simulink model "Paper_Simulation"  (R2020a)
settings: Solver=VariableStepAuto  StartTime=0.0  StopTime=10.0  RelTol=1e-3
model workspace (MAT data in the model file):
  Wo = 1
undefined symbols (not defined in the file): fdesignblkfcn, gcbh, T1, T2, Tf
libraries: eeSinusoidalMeasurementV2 x1, simulink x1
settings Model: Creator=Ayush Agrawal  LastModifiedBy=Ayush Agrawal

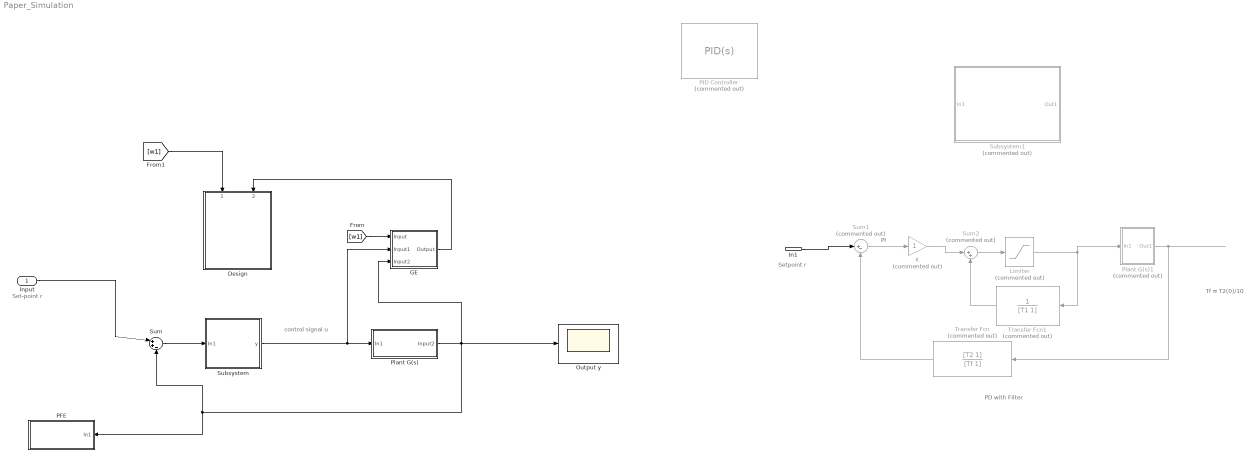
== system Paper_Simulation ==
  note: control signal
      |         u
  note: Set-point r
  note: Setpoint r
  note: PI
  note: PD with Filter
  note: Tf = T2(0)/10
  Input : Inport
  In1 : Inport  Port=2
  Design : Subsystem  mask{a=1.5}
  GE : Subsystem
  K : Gain  Commented=on
  Limiter : Saturate  Commented=on
  Output y : Scope
  PFE : Subsystem
  PID Controller : simulink/Continuous/PID Controller  Commented=on  Controller=PID  Form=Parallel  TimeDomain=Continuous-time  UseExternalTs=off  SampleTime=-1  IntegratorMethod=Forward Euler  FilterMethod=Forward Euler  ControllerParametersSource=internal  P=1  I=1  D=0  UseFilter=on  N=100  TunerSelectOption=Transfer Function Based (PID Tuner App)  InitialConditionSource=internal  InitialConditionForIntegrator=0  InitialConditionForFilter=0  DifferentiatorICPrevScaledInput=0  ExternalReset=none  TrackingMode=off  Kt=1  LimitOutput=off  UpperSaturationLimit=inf  LowerSaturationLimit=-inf  LinearizeAsGain=on  AntiWindupMode=none  Kb=1  POutMin=[]  POutMax=[]  IOutMin=[]  IOutMax=[]  DOutMin=[]  DOutMax=[]  NOutMin=[]  NOutMax=[]  SumOutMin=[]  SumOutMax=[]  SaturationOutMin=[]  SaturationOutMax=[]  PParamMin=[]  PParamMax=[]  IParamMin=[]  IParamMax=[]  DParamMin=[]  DParamMax=[]  NParamMin=[]  NParamMax=[]  KbParamMin=[]  KbParamMax=[]  KtParamMin=[]  KtParamMax=[]  KbOutMin=[]  KbOutMax=[]  KtOutMin=[]  KtOutMax=[]  IntegratorOutMin=[]  IntegratorOutMax=[]  FilterOutMin=[]  FilterOutMax=[]  SumI1OutMin=[]  SumI1OutMax=[]  SumI2OutMin=[]  SumI2OutMax=[]  SumI3OutMin=[]  SumI3OutMax=[]  SumI4OutMin=[]  SumI4OutMax=[]  SumDOutMin=[]  SumDOutMax=[]  DifferentiatorOutMin=[]  DifferentiatorOutMax=[]  FilterDiffOutCoefMin=[]  FilterDiffOutCoefMax=[]  ReciprocalOutMin=[]  ReciprocalOutMax=[]  SumDenOutMin=[]  SumDenOutMax=[]  SumNumOutMin=[]  SumNumOutMax=[]  DivideOutMin=[]  DivideOutMax=[]  UdiffTsProdOutMin=[]  UdiffTsProdOutMax=[]  NTsProdOutMin=[]  NTsProdOutMax=[]  UintegralTsProdOutMin=[]  UintegralTsProdOutMax=[]  UngainTsProdOutMin=[]  UngainTsProdOutMax=[]  IntegratorContinuousStateAttributes=''  IntegratorStateMustResolveToSignalObject=off  IntegratorRTWStateStorageClass=Auto  FilterContinuousStateAttributes=''  FilterStateMustResolveToSignalObject=off  FilterRTWStateStorageClass=Auto  ParallelPVariant=InternalParameters  IdealPVariant=Disabled  IVariant=InternalParameters  DVariant=InternalParameters  IntegratorVariant=Continuous  SatVariant=Disabled  AWVariant=Passthrough  PCopyVariant=Disabled  TRVariant=Disabled  FdbkBlocksVariant=Forward  IdealPFdbkVariant=Disabled  SatFdbkVariant=Disabled  DerivativeFilterVariant=ContFilter  NVariant=InternalParameters  NCopyVariant=Disabled  FilterICVariant=InternalICsFilter  IntegratorICVariant=InternalICs  ExternalResetVariant=Disabled  TRSumVariant=Passthrough  SumFdbkVariant=Disabled  SumVariant=Sum_PID  TsampFilterVariant=InternalTs  TsampNgainVariant=Passthrough  TsampIntegralVariant=Passthrough
  Plant G(s) : Subsystem
  Plant G(s)1 : Subsystem  Commented=on
  Subsystem : Subsystem  mask{Ti=0, r=0}
  Subsystem1 : Subsystem  Commented=on
  Sum : Sum  Inputs=|++-
  Sum1 : Sum  Commented=on  Inputs=|+-
  Sum2 : Sum  Commented=on  Inputs=|++
  Transfer Fcn : TransferFcn  Commented=on  Numerator=[T2 1]  Denominator=[Tf 1]
  Transfer Fcn1 : TransferFcn  Commented=on  Denominator=[T1 1]
  wires:
  Plant G(s)/1(Input2) -> GE/3(Input2), Output y/1, Sum/3, PFE/1(In1)
  ? -> Sum/2
  Input/1 -> Sum/1
  Sum2/1 -> Limiter/1
  In1/1 -> Sum1/1
  Plant G(s)1/1(Out1) -> Transfer Fcn/1
  Limiter/1 -> Transfer Fcn1/1, Plant G(s)1/1(In1)
  Sum1/1 -> K/1
  Transfer Fcn/1 -> Sum1/2
  K/1 -> Sum2/1
  Transfer Fcn1/1 -> Sum2/2
  [w1] -> GE/1(Input)
  GE/1(Output) -> Design/2(Plant Gain Amplitude)
  [w1] -> Design/1(PFE O/P frequency)
  Subsystem/1(y) -> GE/2(Input1), Plant G(s)/1(In1)
  Sum/1 -> Subsystem/1(In1)

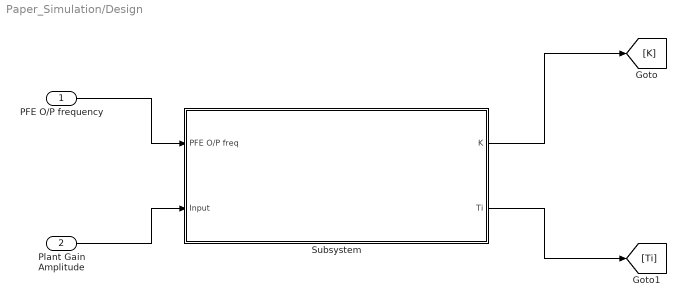
== system Paper_Simulation/Design ==
  PFE O/P frequency : Inport
  Plant Gain Amplitude : Inport  Port=2
  Subsystem : Subsystem
  wires:
  PFE O/P frequency/1 -> Subsystem/1(PFE O/P freq)
  Plant Gain Amplitude/1 -> Subsystem/2(Input)
  Subsystem/1(K) -> [K]
  Subsystem/2(Ti) -> [Ti]

== system Paper_Simulation/GE ==
  Input : Inport
  Input1 : Inport  Port=2
  Input2 : Inport  Port=3
  Amplitude Estimator : Subsystem
  Output : Outport
  wires:
  Input1/1 -> Amplitude Estimator/1(In1)
  Input/1 -> Amplitude Estimator/2(Input)
  Amplitude Estimator/1(Output) -> Output/1

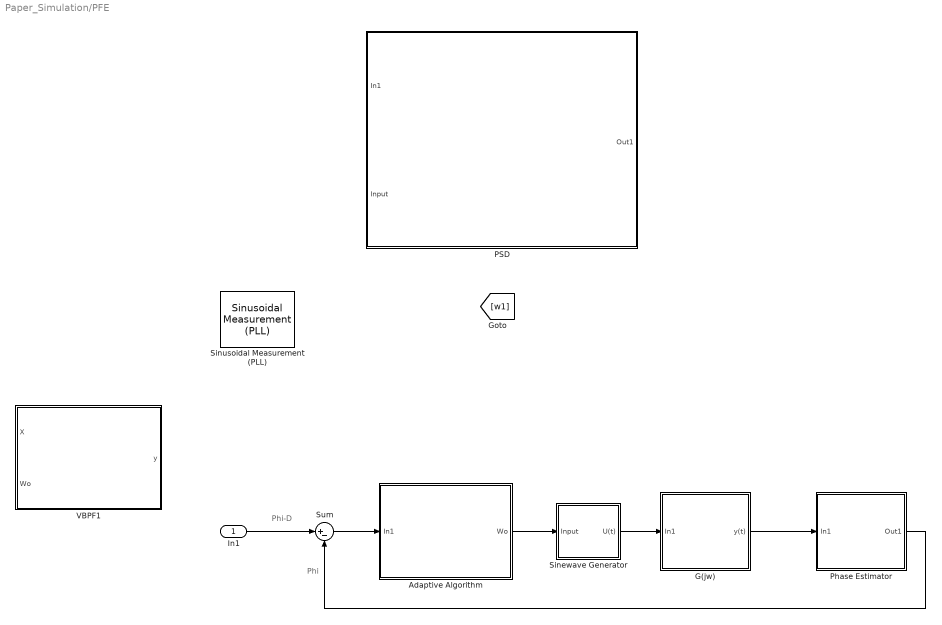
== system Paper_Simulation/PFE ==
  note: Phi
  note: Phi-D
  In1 : Inport
  Adaptive Algorithm : Subsystem
  G(jw) : Subsystem
  PSD : Subsystem
  Phase Estimator : Subsystem
  Sinewave Generator : Subsystem
  Sinusoidal Measurement (PLL) : eeSinusoidalMeasurementV2/Sinusoidal Measurement (PLL)  Ki_PD=1000  Kp_LF=400  Ki_LF=20000  F0=60  Theta0=0  Mag0=1  Ts=-1
      settings: SourceProductBaseCode=PS
  Sum : Sum  Inputs=|+-
  VBPF1 : Subsystem
  wires:
  In1/1 -> Sum/1
  Sum/1 -> Adaptive Algorithm/1(In1)
  Adaptive Algorithm/1(Wo) -> Sinewave Generator/1(Input)
  Sinewave Generator/1(U(t)) -> G(jw)/1(In1)
  G(jw)/1(y(t)) -> Phase Estimator/1(In1)
  Phase Estimator/1(Out1) -> Sum/2

== system Paper_Simulation/Plant G(s) ==
  In1 : Inport
  Input2 : Outport
  wires:
  In1/1 -> Input2/1

== system Paper_Simulation/Plant G(s)1 ==
  In1 : Inport
  Out1 : Outport
  wires:
  In1/1 -> Out1/1

== system Paper_Simulation/Subsystem ==
  In1 : Inport
  Controller : Subsystem  mask{Td=Ti*r, Tf=0, T1=Ti/2, T2=Ti/2}
  y : Outport
  wires:
  Controller/1(y) -> y/1
  In1/1 -> Controller/1(In1)

== system Paper_Simulation/Subsystem1 ==
  In1 : Inport
  Out1 : Outport
  wires:
  In1/1 -> Out1/1

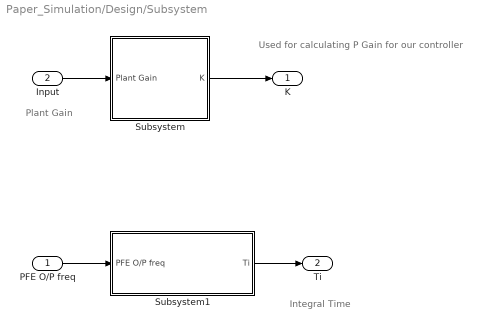
== system Paper_Simulation/Design/Subsystem ==
  note: Used for calculating P Gain for our controller
  note: Integral Time
  note: Plant Gain
  PFE O/P freq : Inport
  Input : Inport  Port=2
  Subsystem : Subsystem
  Subsystem1 : Subsystem
  K : Outport
  Ti : Outport  Port=2
  wires:
  Input/1 -> Subsystem/1(Plant Gain)
  Subsystem/1(K) -> K/1
  PFE O/P freq/1 -> Subsystem1/1(PFE O/P freq)
  Subsystem1/1(Ti) -> Ti/1

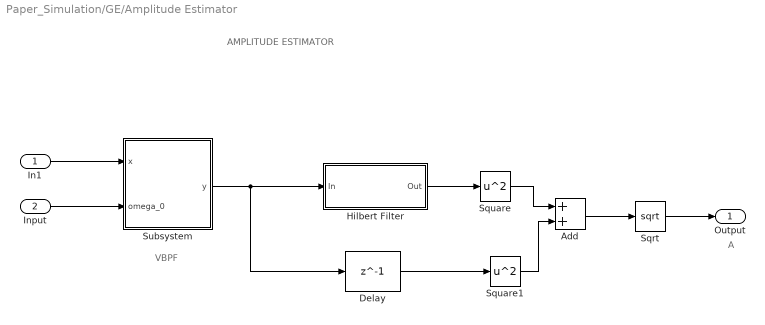
== system Paper_Simulation/GE/Amplitude Estimator ==
  note: A
  note: AMPLITUDE ESTIMATOR
  note: VBPF
  In1 : Inport
  Input : Inport  Port=2
  Add : Sum
  Delay : Delay  DelayLength=1  InitialCondition=0  UseCircularBuffer=on
  Hilbert Filter : Subsystem  DialogController=fdesignblkfcn  InitFcn=fdesignblkfcn(gcbh, {'InitFcn'});  mask(Hilbert Filter){}
      mask help: Design a Hilbert filter
      settings: CopyFcn=fdesignblkfcn(gcbh, {'CopyFcn'});
      mask Help: helpview(mapfilelocation('dsp'), 'dsphilbertfilter');
      mask Display: disp('Hilbert')
  Sqrt : Sqrt  SaturateOnIntegerOverflow=on
  Square : Math  Operator=square  SaturateOnIntegerOverflow=on
  Square1 : Math  Operator=square  SaturateOnIntegerOverflow=on
  Subsystem : Subsystem
  Output : Outport
  wires:
  Input/1 -> Subsystem/2(omega_0)
  In1/1 -> Subsystem/1(x)
  Subsystem/1(y) -> Delay/1, Hilbert Filter/1(In)
  Hilbert Filter/1(Out) -> Square/1
  Delay/1 -> Square1/1
  Square/1 -> Add/1
  Square1/1 -> Add/2
  Add/1 -> Sqrt/1
  Sqrt/1 -> Output/1

== system Paper_Simulation/PFE/Adaptive Algorithm ==
  In1 : Inport
  Wo : Outport
  wires:
  In1/1 -> Wo/1

== system Paper_Simulation/PFE/G(jw) ==
  In1 : Inport
  y(t) : Outport

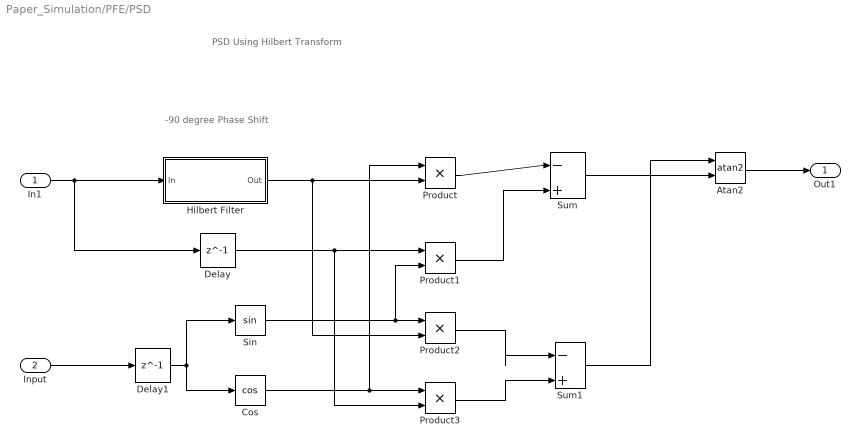
== system Paper_Simulation/PFE/PSD ==
  note: -90 degree Phase Shift
  note: PSD Using Hilbert Transform
  In1 : Inport
  Input : Inport  Port=2
  Atan2 : Trigonometry  Operator=atan2
  Cos : Trigonometry  Operator=cos
  Delay : Delay  DelayLength=1
  Delay1 : Delay  DelayLength=1
  Hilbert Filter : Subsystem  DialogController=fdesignblkfcn  InitFcn=fdesignblkfcn(gcbh, {'InitFcn'});  mask(Hilbert Filter){}
      mask help: Design a Hilbert filter
      settings: CopyFcn=fdesignblkfcn(gcbh, {'CopyFcn'});
      mask Help: helpview(mapfilelocation('dsp'), 'dsphilbertfilter');
      mask Display: disp('Hilbert')
  Product{,1..3} (4 alike) : Product
  Sin : Trigonometry
  Sum : Sum  Inputs=|-+
  Sum1 : Sum  Inputs=|-+
  Out1 : Outport
  wires:
  In1/1 -> Delay/1, Hilbert Filter/1(In)
  Hilbert Filter/1(Out) -> Product2/2, Product/2
  Input/1 -> Delay1/1
  Delay1/1 -> Sin/1, Cos/1
  Sin/1 -> Product1/2, Product2/1
  Cos/1 -> Product/1, Product3/1
  Delay/1 -> Product3/2, Product1/1
  Product/1 -> Sum/1
  Product1/1 -> Sum/2
  Atan2/1 -> Out1/1
  Sum/1 -> Atan2/2
  Product2/1 -> Sum1/1
  Product3/1 -> Sum1/2
  Sum1/1 -> Atan2/1

== system Paper_Simulation/PFE/Phase Estimator ==
  In1 : Inport
  Out1 : Outport
  wires:
  In1/1 -> Out1/1

== system Paper_Simulation/PFE/Sinewave Generator ==
  Input : Inport
  U(t) : Outport

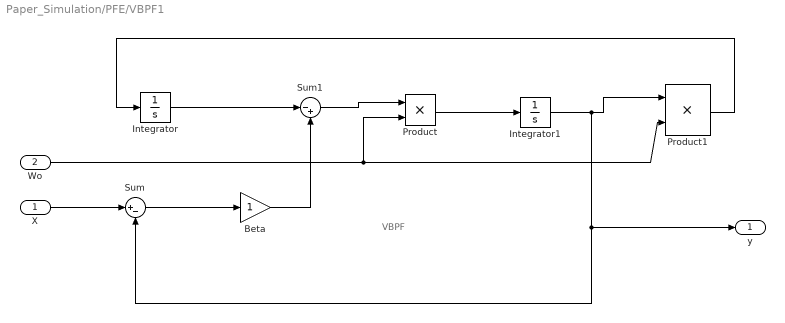
== system Paper_Simulation/PFE/VBPF1 ==
  note: VBPF
  X : Inport
  Wo : Inport  Port=2
  Beta : Gain
  Integrator : Integrator
  Integrator1 : Integrator
  Product : Product
  Product1 : Product
  Sum : Sum  Inputs=|+-
  Sum1 : Sum  Inputs=|-+
  y : Outport
  wires:
  X/1 -> Sum/1
  Sum/1 -> Beta/1
  Integrator/1 -> Sum1/1
  Beta/1 -> Sum1/2
  Sum1/1 -> Product/1
  Wo/1 -> Product1/2, Product/2
  Product/1 -> Integrator1/1
  Integrator1/1 -> Product1/1, Sum/2, y/1
  Product1/1 -> Integrator/1

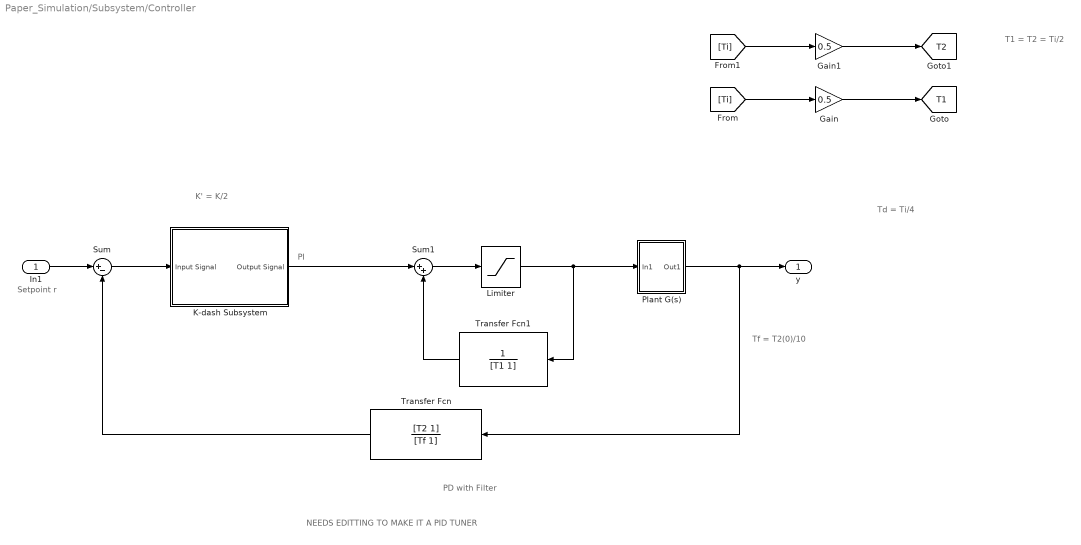
== system Paper_Simulation/Subsystem/Controller ==
  note: K' = K/2
  note: Td = Ti/4
  note: T1 = T2 = Ti/2
  note: NEEDS EDITTING TO MAKE IT A PID TUNER
  note: PI
  note: PD with Filter
  note: Setpoint r
  note: Tf = T2(0)/10
  In1 : Inport
  Gain : Gain  Gain=0.5
  Gain1 : Gain  Gain=0.5
  K-dash Subsystem : Subsystem
  Limiter : Saturate
  Plant G(s) : Subsystem
  Sum : Sum  Inputs=|+-
  Sum1 : Sum  Inputs=|++
  Transfer Fcn : TransferFcn  Numerator=[T2 1]  Denominator=[Tf 1]
  Transfer Fcn1 : TransferFcn  Denominator=[T1 1]
  y : Outport
  tag scope: T1=global, T2=global
  wires:
  Sum/1 -> K-dash Subsystem/1(Input Signal)
  Sum1/1 -> Limiter/1
  Limiter/1 -> Transfer Fcn1/1, Plant G(s)/1(In1)
  Transfer Fcn1/1 -> Sum1/2
  In1/1 -> Sum/1
  K-dash Subsystem/1(Output Signal) -> Sum1/1
  Plant G(s)/1(Out1) -> Transfer Fcn/1, y/1
  Transfer Fcn/1 -> Sum/2
  [Ti] -> Gain/1
  Gain/1 -> [T1]
  Gain1/1 -> [T2]
  [Ti] -> Gain1/1

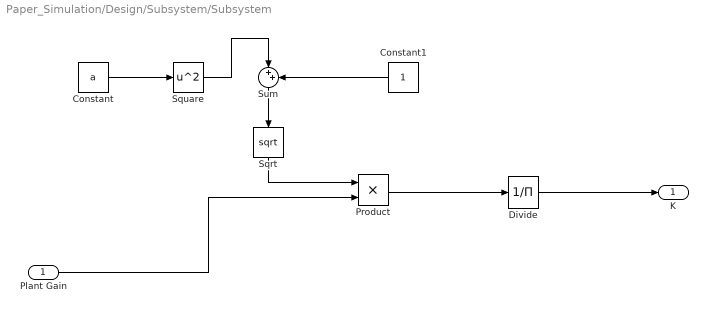
== system Paper_Simulation/Design/Subsystem/Subsystem ==
  Plant Gain : Inport
  Constant : Constant  Value=a
  Constant1 : Constant
  Divide : Product  Inputs=/
  Product : Product
  Sqrt : Sqrt  SaturateOnIntegerOverflow=on
  Square : Math  Operator=square  SaturateOnIntegerOverflow=on
  Sum : Sum  Inputs=|++
  K : Outport
  wires:
  Divide/1 -> K/1
  Sum/1 -> Sqrt/1
  Square/1 -> Sum/1
  Sqrt/1 -> Product/1
  Plant Gain/1 -> Product/2
  Constant/1 -> Square/1
  Product/1 -> Divide/1
  Constant1/1 -> Sum/2

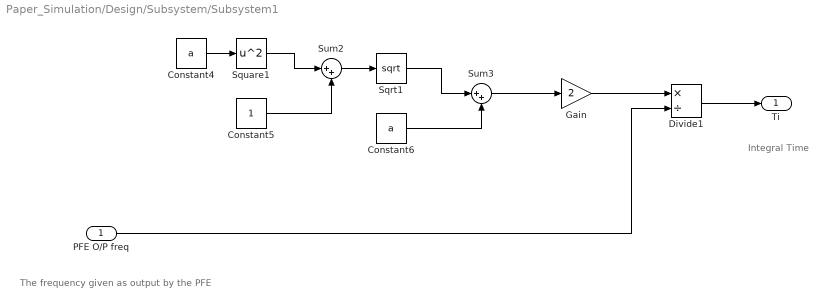
== system Paper_Simulation/Design/Subsystem/Subsystem1 ==
  note: Integral Time
  note: The frequency given as output by the PFE
  PFE O/P freq : Inport
  Constant4 : Constant  Value=a
  Constant5 : Constant
  Constant6 : Constant  Value=a
  Divide1 : Product  Inputs=*/
  Gain : Gain  Gain=2
  Sqrt1 : Sqrt  SaturateOnIntegerOverflow=on
  Square1 : Math  Operator=square  SaturateOnIntegerOverflow=on
  Sum2 : Sum  Inputs=|++
  Sum3 : Sum  Inputs=|++
  Ti : Outport
  wires:
  Constant6/1 -> Sum3/2
  PFE O/P freq/1 -> Divide1/2
  Sum3/1 -> Gain/1
  Gain/1 -> Divide1/1
  Sum2/1 -> Sqrt1/1
  Constant5/1 -> Sum2/2
  Constant4/1 -> Square1/1
  Sqrt1/1 -> Sum3/1
  Square1/1 -> Sum2/1
  Divide1/1 -> Ti/1

== system Paper_Simulation/GE/Amplitude Estimator/Hilbert Filter ==
  In : Inport
  Generated Filter Block : DiscreteFir  Tag=BlockMethodSubSystem  Coefficients=[-0.026449858259791379 -0.00578355491829027 -0.016572261903348456 -0.0095390561131982743 -0.022461390535071568 -0.014999256435125952 -0.030323967074738556 -0.023012528163449009 -0.041429315821655127 -0.035762828939278346 -0.05911752381753177 -0.059034685410808696 -0.094459906652176406 -0.11739830204172252 -0.21797718993610349 -0.62869353747279177 0.62869353747279177 0.21797718993610349 0.11739830204172252 0.094459906652176406 0.059034685410808696 0.05911752381753177 0.035762828939278346 0.041429315821655127 0.023012528163449009 0.030323967074738556 0.014999256435125952 0.022461390535071568 0.0095390561131982743 0.016572261903348456 0.00578355491829027 0.026449858259791379]  InputProcessing=Columns as channels (frame based)
  Out : Outport  VectorParamsAs1DForOutWhenUnconnected=off
  wires:
  Generated Filter Block/1 -> Out/1
  In/1 -> Generated Filter Block/1

== system Paper_Simulation/GE/Amplitude Estimator/Subsystem ==
  x : Inport
  omega_0 : Inport  Port=2
  VBPF : Subsystem
  y : Outport
  wires:
  omega_0/1 -> VBPF/2(Wo)
  x/1 -> VBPF/1(X)
  VBPF/1(y) -> y/1

== system Paper_Simulation/PFE/PSD/Hilbert Filter ==
  In : Inport
  Generated Filter Block : DiscreteFir  Tag=BlockMethodSubSystem  Coefficients=[-0.026449858259791379 -0.00578355491829027 -0.016572261903348456 -0.0095390561131982743 -0.022461390535071568 -0.014999256435125952 -0.030323967074738556 -0.023012528163449009 -0.041429315821655127 -0.035762828939278346 -0.05911752381753177 -0.059034685410808696 -0.094459906652176406 -0.11739830204172252 -0.21797718993610349 -0.62869353747279177 0.62869353747279177 0.21797718993610349 0.11739830204172252 0.094459906652176406 0.059034685410808696 0.05911752381753177 0.035762828939278346 0.041429315821655127 0.023012528163449009 0.030323967074738556 0.014999256435125952 0.022461390535071568 0.0095390561131982743 0.016572261903348456 0.00578355491829027 0.026449858259791379]  InputProcessing=Columns as channels (frame based)
  Out : Outport  VectorParamsAs1DForOutWhenUnconnected=off
  wires:
  Generated Filter Block/1 -> Out/1
  In/1 -> Generated Filter Block/1

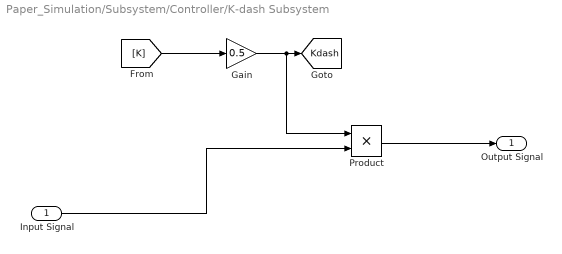
== system Paper_Simulation/Subsystem/Controller/K-dash Subsystem ==
  Input Signal : Inport
  Gain : Gain  Gain=0.5
  Product : Product
  Output Signal : Outport
  tag scope: Kdash=global
  wires:
  Gain/1 -> Product/1, [Kdash]
  [K] -> Gain/1
  Input Signal/1 -> Product/2
  Product/1 -> Output Signal/1

== system Paper_Simulation/Subsystem/Controller/Plant G(s) ==
  In1 : Inport
  Out1 : Outport
  wires:
  In1/1 -> Out1/1

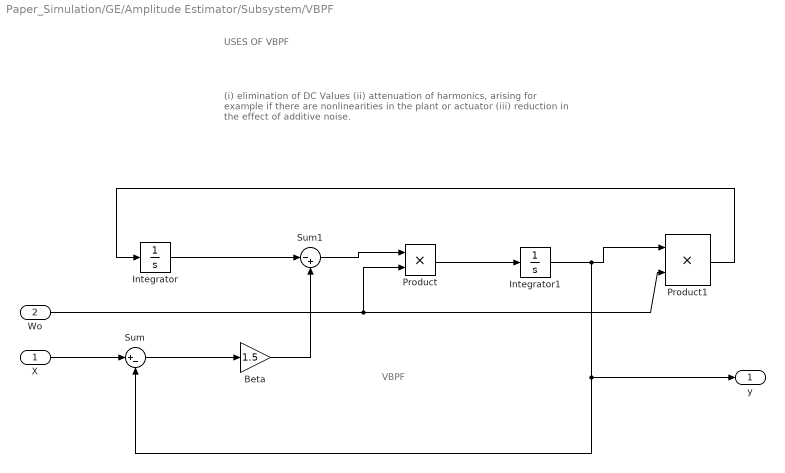
== system Paper_Simulation/GE/Amplitude Estimator/Subsystem/VBPF ==
  note: USES OF VBPF
  note: (i) elimination of DC Values
      | (ii) attenuation of harmonics, arising for example if there
      | are nonlinearities in the plant or actuator
      | (iii) reduction in the effect of additive noise.
  note: VBPF
  X : Inport
  Wo : Inport  Port=2
  Beta : Gain  Gain=1.5
  Integrator : Integrator
  Integrator1 : Integrator
  Product : Product
  Product1 : Product
  Sum : Sum  Inputs=|+-
  Sum1 : Sum  Inputs=|-+
  y : Outport
  wires:
  X/1 -> Sum/1
  Sum/1 -> Beta/1
  Integrator/1 -> Sum1/1
  Beta/1 -> Sum1/2
  Sum1/1 -> Product/1
  Wo/1 -> Product1/2, Product/2
  Product/1 -> Integrator1/1
  Integrator1/1 -> Product1/1, Sum/2, y/1
  Product1/1 -> Integrator/1
